simulink model "Ellipse"  (R2023b)
settings: Solver=FixedStepAuto  StartTime=0.0  StopTime=10.0  RelTol=1e-3
settings Model: Creator=Eric  LastModifiedBy=no
settings SolverCC: AlgebraicLoopSolver=LineSearch
settings DataIOCC: SaveOutput=off  ReturnWorkspaceOutputs=off
settings OptimizationCC: DefaultParameterBehavior=Inlined
settings DebuggingCC: UnconnectedInputMsg=warning  UnconnectedOutputMsg=warning  UnconnectedLineMsg=warning  ArithmeticOperatorsInVariantConditions=warning
settings ModelReferenceCC: EnableRefExpFcnMdlSchedulingChecks=on
settings SFSimCC: SimUseLocalCustomCode=off  CustomCodeUndefinedFunction=UseInterfaceOnly
settings RTWCC: Description=INTECRIO Real-Time Target  SystemTargetFile=irt.tlc  TemplateMakefile=irt_default_tmf  RTWUseLocalCustomCode=off
settings STFCustomTargetCC: UtilityFuncGeneration=Shared location  MatFileLogging=on  GRTInterface=on  SystemTargetFile=irt.tlc
settings GRTTargetCC: UtilityFuncGeneration=Shared location  ParMdlRefBuildCompliant=off  CompOptLevelCompliant=off  ConcurrentExecutionCompliant=off  CombineOutputUpdateFcns=off  CPPClassGenCompliant=off  GRTInterface=on  UseToolchainInfoCompliant=off  GenerateASAP2=on

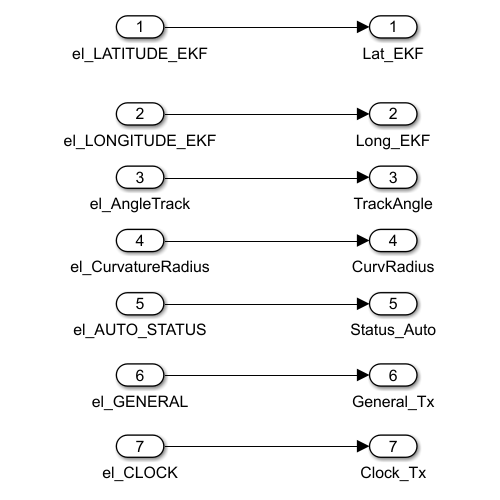
[thumbnail: Simulink's stored preview of the top-level diagram]
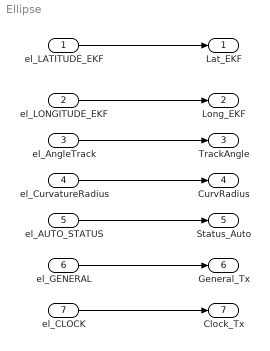
== system Ellipse ==
  el_LATITUDE_EKF : Inport
  el_LONGITUDE_EKF : Inport  Port=2
  el_AngleTrack : Inport  Port=3
  el_CurvatureRadius : Inport  Port=4
  el_AUTO_STATUS : Inport  Port=5
  el_GENERAL : Inport  Port=6
  el_CLOCK : Inport  Port=7
  Lat_EKF : Outport  VectorParamsAs1DForOutWhenUnconnected=off
  Long_EKF : Outport  Port=2  VectorParamsAs1DForOutWhenUnconnected=off
  TrackAngle : Outport  Port=3  VectorParamsAs1DForOutWhenUnconnected=off
  CurvRadius : Outport  Port=4  VectorParamsAs1DForOutWhenUnconnected=off
  Status_Auto : Outport  Port=5  VectorParamsAs1DForOutWhenUnconnected=off
  General_Tx : Outport  Port=6  VectorParamsAs1DForOutWhenUnconnected=off
  Clock_Tx : Outport  Port=7  VectorParamsAs1DForOutWhenUnconnected=off
  wires:
  el_CLOCK/1 -> Clock_Tx/1
  el_GENERAL/1 -> General_Tx/1
  el_AUTO_STATUS/1 -> Status_Auto/1
  el_CurvatureRadius/1 -> CurvRadius/1
  el_AngleTrack/1 -> TrackAngle/1
  el_LONGITUDE_EKF/1 -> Long_EKF/1
  el_LATITUDE_EKF/1 -> Lat_EKF/1
